simulink model "swpwmctrl"  (Simulink 7.0)
settings: Solver=ode1  StartTime=0.0  StopTime=4  FixedStep=0.0002  RelTol=1e-3
undefined symbols (not defined in the file or in its folder): Model_626, Sensoray
libraries: rtwinlib x6, simulink x6, dsparch4 x5, dspsigops x2, dspswit3 x2
settings Model: Creator=user  LastModifiedBy=user_2  SimulationMode=external  ExtModeTrigDuration=60000  BufferReuse=off
settings SolverCC: PositivePriorityOrder=on
settings DataIOCC: MaxDataPoints=60000
settings OptimizationCC: BooleanDataType=off  InlineInvariantSignals=on  OptimizeBlockIOStorage=off  BufferReuse=off  ExpressionFolding=off  LocalBlockOutputs=off
settings HardwareCC: TargetEndianess=LittleEndian  TargetHWDeviceType=MATLAB Host
settings RTWCC: SystemTargetFile=rtwin.tlc  TemplateMakefile=rtwin.tmf  Description=Real-Time Windows Target  ProcessScript=rtwin_make_rtw_hook
settings RTWinTargetCC: GenFloatMathFcnCalls=ANSI_C  ModelReferenceCompliant=off  CompOptLevelCompliant=off  PortableWordSizes=off  CCOptimize=on

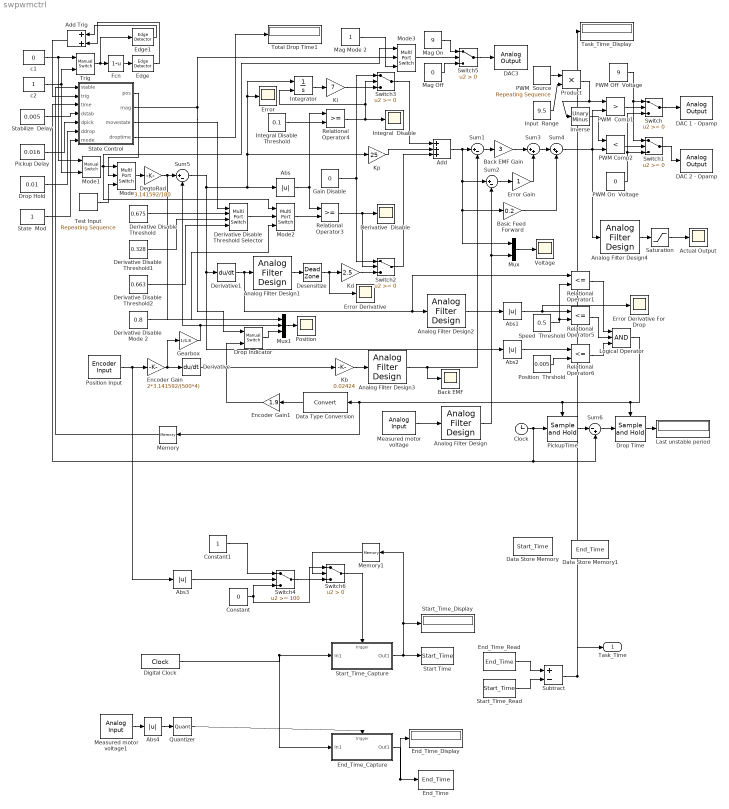
== system swpwmctrl ==
  Abs{,1..4} (5 alike) : Abs  OutDataType=sfix(16)  OutScaling=2^0
  Actual Output : Scope
      settings: YMin=-15  YMax=15  SaveName=ScopeData4  MaxDataPoints=60000
  Add : Sum  Inputs=+++  OutDataType=sfix(16)  OutScaling=2^-10
  Add Trig : Sum  Orientation=left  OutDataType=sfix(16)  OutScaling=2^-10
  Analog Filter Design : dsparch4/Analog Filter Design  method=Butterworth  filttype=Lowpass  N=3  Wlo=100  Whi=80  Rp=2  Rs=40
  Analog Filter Design1 : dsparch4/Analog Filter Design  method=Butterworth  filttype=Lowpass  N=3  Wlo=100  Whi=80  Rp=2  Rs=40
  Analog Filter Design2 : dsparch4/Analog Filter Design  method=Butterworth  filttype=Lowpass  N=3  Wlo=80  Whi=80  Rp=2  Rs=40
  Analog Filter Design3 : dsparch4/Analog Filter Design  method=Butterworth  filttype=Lowpass  N=3  Wlo=100  Whi=80  Rp=2  Rs=40
  Analog Filter Design4 : dsparch4/Analog Filter Design  method=Butterworth  filttype=Lowpass  N=3  Wlo=85  Whi=80  Rp=2  Rs=40
  Back EMF : Scope
      settings: YMin=-1  YMax=1  SaveName=ScopeData10  MaxDataPoints=60000
  Back EMF Gain : Gain  Gain=3  ParameterDataType=sfix(16)  ParameterScaling=2^0  OutDataType=sfix(16)  OutScaling=2^0
  Basic Feed  Forward : Gain  Gain=0.2  ParameterDataType=sfix(16)  ParameterScaling=2^0  OutDataType=sfix(16)  OutScaling=2^0
  Clock : Clock
      settings: Decimation=10
  Constant : Constant  Value=0  OutDataType=sfix(16)  OutScaling=2^0
  Constant1 : Constant  OutDataType=sfix(16)  OutScaling=2^0
  DAC 1 - Opamp : rtwinlib/Analog Output  SampleTime=-1  DrvName=Sensoray/Model_626  DrvAddress=4294967295  DrvOptions=zeros(1,0)  Channels=1  RangeMode=1  VoltRange=1  InitialValue=[]  FinalValue=[]
      settings: AttributesFormatString=Sensoray\nModel 626 [auto]
  DAC 2 - Opamp : rtwinlib/Analog Output  SampleTime=-1  DrvName=Sensoray/Model_626  DrvAddress=4294967295  DrvOptions=zeros(1,0)  Channels=2  RangeMode=1  VoltRange=1  InitialValue=[]  FinalValue=[]
      settings: AttributesFormatString=Sensoray\nModel 626 [auto]
  DAC3 : rtwinlib/Analog Output  SampleTime=-1  DrvName=Sensoray/Model_626  DrvAddress=4294967295  DrvOptions=zeros(1,0)  Channels=3  RangeMode=1  VoltRange=1  InitialValue=[]  FinalValue=[]
      settings: AttributesFormatString=Sensoray\nModel 626 [auto]
  Data Store Memory : DataStoreMemory  DataStoreName=Start_Time  ReadBeforeWriteMsg=warning  WriteAfterWriteMsg=warning  WriteAfterReadMsg=warning  OutDataType=sfix(16)  OutScaling=2^0
  Data Store Memory1 : DataStoreMemory  DataStoreName=End_Time  ReadBeforeWriteMsg=warning  WriteAfterWriteMsg=warning  WriteAfterReadMsg=warning  OutDataType=sfix(16)  OutScaling=2^0
  Data Type Conversion : DataTypeConversion  Orientation=left  OutDataTypeMode=double  OutDataType=sfix(16)  OutScaling=2^0
  DegtoRad : Gain  Gain=3.141592/180  ParameterDataType=sfix(16)  ParameterScaling=2^0  OutDataType=sfix(16)  OutScaling=2^0
  Derivative : Derivative
  Derivative  Disable : Scope
      settings: YMin=-0.25  YMax=3.25  SaveName=ScopeData3  MaxDataPoints=60000
  Derivative Disable Mode 2 : Constant  Value=0.8  OutDataType=sfix(16)  OutScaling=2^0
  Derivative Disable Threshold : Constant  Value=0.675  OutDataType=sfix(16)  OutScaling=2^0
  Derivative Disable Threshold Selector : MultiPortSwitch  Inputs=3  zeroidx=on  OutDataType=sfix(16)  OutScaling=2^0
  Derivative Disable Threshold1 : Constant  Value=0.328  OutDataType=sfix(16)  OutScaling=2^0
  Derivative Disable Threshold2 : Constant  Value=0.663  OutDataType=sfix(16)  OutScaling=2^0
  Derivative1 : Derivative
  Desensitize : DeadZone  LowerValue=-0.1  UpperValue=0.1  SaturateOnIntegerOverflow=on
  Digital Clock : DigitalClock  SampleTime=-1
  Drop Hold : Constant  Value=0.01  OutDataType=sfix(16)  OutScaling=2^0
  Drop Indicator : simulink/Signal Routing/Manual Switch  SystemSampleTime=-1  sw=1  action=0  varsize=off
  Drop Time : dspsigops/Sample and Hold  SystemSampleTime=-1  trig=Rising edge  initCond=0  latchinput=off
  Edge : dspswit3/Edge Detector  SystemSampleTime=-1
  Edge1 : dspswit3/Edge Detector  SystemSampleTime=-1
  Encoder Gain : Gain  Gain=2*3.141592/(500*4)  ParameterDataType=sfix(16)  ParameterScaling=2^0  OutDataType=sfix(16)  OutScaling=2^0
  Encoder Gain1 : Gain  Orientation=left  Gain=1.9  ParameterDataType=sfix(16)  ParameterScaling=2^0  OutDataType=sfix(16)  OutScaling=2^0
  End_Time : DataStoreWrite  DataStoreName=End_Time  SampleTime=-1
  End_Time_Capture : Subsystem  TreatAsAtomicUnit=on
  End_Time_Display : Display
  End_Time_Read : DataStoreRead  DataStoreName=End_Time  SampleTime=0
  Error : Scope
      settings: YMin=-0.05  YMax=0.05  SaveName=ScopeData2  MaxDataPoints=60000
  Error Derivative : Scope
      settings: YMin=-1  YMax=1  SaveName=ScopeData8  MaxDataPoints=60000
  Error Derivative For Drop : Scope
      settings: YMin=0  YMax=2  SaveName=ScopeData9  MaxDataPoints=60000
  Error Gain : Gain  ParameterDataType=sfix(16)  ParameterScaling=2^0  OutDataType=sfix(16)  OutScaling=2^0
  Fcn : Fcn  Expr=1-u
  Gain Disable : Constant  Value=0  OutDataType=sfix(16)  OutScaling=2^0
  Gearbox : Gain  Gain=1/4.8  ParameterDataType=sfix(16)  ParameterScaling=2^0  OutDataType=sfix(16)  OutScaling=2^0
  Input  Range : Constant  Value=9.5  OutDataType=sfix(16)  OutScaling=2^0
  Integral  Disable : Scope
      settings: YMin=-0.25  YMax=3.25  SaveName=ScopeData5  MaxDataPoints=60000
  Integral Disable Threshold : Constant  Value=0.1  OutDataType=sfix(16)  OutScaling=2^0
  Integrator : Integrator  ExternalReset=falling
  Inverse : simulink/Math Operations/Unary Minus  DoSatur=off
  Kb : Gain  Gain=0.02424  ParameterDataType=sfix(16)  ParameterScaling=2^0  OutDataType=sfix(16)  OutScaling=2^0
  Kd : Gain  Gain=2.5  ParameterDataType=sfix(16)  ParameterScaling=2^0  OutDataType=sfix(16)  OutScaling=2^0
  Ki : Gain  Gain=7  ParameterDataType=sfix(16)  ParameterScaling=2^0  OutDataType=sfix(16)  OutScaling=2^0
  Kp : Gain  Gain=25  ParameterDataType=sfix(16)  ParameterScaling=2^0  OutDataType=sfix(16)  OutScaling=2^0
  Last unstable period : Display
  Logical Operator : Logic  Inputs=3  AllPortsSameDT=off  OutDataTypeMode=boolean
  Mag Mode 2 : Constant  OutDataType=sfix(16)  OutScaling=2^0
  Mag Off : Constant  Value=0  OutDataType=sfix(16)  OutScaling=2^0
  Mag On : Constant  Value=9  OutDataType=sfix(16)  OutScaling=2^0
  Measured motor voltage : rtwinlib/Analog Input  SampleTime=-1  DrvName=Sensoray/Model_626  DrvAddress=4294967295  DrvOptions=zeros(1,0)  Channels=1  RangeMode=1  VoltRange=1  DataType=1
      settings: AttributesFormatString=Sensoray\nModel 626 [auto]
  Measured motor voltage1 : rtwinlib/Analog Input  SampleTime=-1  DrvName=Sensoray/Model_626  DrvAddress=4294967295  DrvOptions=zeros(1,0)  Channels=2  RangeMode=1  VoltRange=1  DataType=1
      settings: AttributesFormatString=Sensoray\nModel 626 [auto]
  Memory : Memory  Orientation=left
  Memory1 : Memory  Orientation=left
  Mode : MultiPortSwitch  Inputs=2  zeroidx=on  OutDataType=sfix(16)  OutScaling=2^0
  Mode1 : simulink/Signal Routing/Manual Switch  SystemSampleTime=-1  sw=1  action=0  varsize=off
  Mode2 : MultiPortSwitch  Inputs=2  zeroidx=on  OutDataType=sfix(16)  OutScaling=2^0
  Mode3 : MultiPortSwitch  Inputs=2  zeroidx=on  OutDataType=sfix(16)  OutScaling=2^0
  Mux : Mux  Inputs=2
  Mux1 : Mux  Inputs=3
  PWM Comp2 : RelationalOperator  Operator=<  LogicOutDataTypeMode=boolean
  PWM  Comp1 : RelationalOperator  Operator=>  LogicOutDataTypeMode=boolean
  PWM  Source : simulink/Sources/Repeating Sequence  SystemSampleTime=-1  rep_seq_t=[0 0.01]  rep_seq_y=[0 1]
  PWM Off  Voltage : Constant  Value=9  OutDataType=sfix(16)  OutScaling=2^0
  PWM On  Voltage : Constant  Value=0  OutDataType=sfix(16)  OutScaling=2^0
  Pickup Delay : Constant  Value=0.016  OutDataType=sfix(16)  OutScaling=2^0
  PickupTime : dspsigops/Sample and Hold  SystemSampleTime=-1  trig=Falling edge  initCond=0  latchinput=off
  Position : Scope
      settings: YMin=-2  YMax=1.2  MaxDataPoints=60000
  Position  Thrshold : Constant  Value=0.005  OutDataType=sfix(16)  OutScaling=2^0
  Position Input : rtwinlib/Encoder Input  SampleTime=-1  DrvName=Sensoray/Model_626  DrvAddress=4294967295  DrvOptions=zeros(1,0)  Channels=[4]  QuadMode=3  IndexPulse=2  InputFilter=Inf  DataType=1
      settings: AttributesFormatString=Sensoray\nModel 626 [auto]
  Product : Product  OutDataType=sfix(16)  OutScaling=2^0  RndMeth=Zero
  Quantizer : Quantizer
  Relational Operator1 : RelationalOperator  Operator=<=  LogicOutDataTypeMode=boolean
  Relational Operator3 : RelationalOperator  LogicOutDataTypeMode=boolean
  Relational Operator4 : RelationalOperator  LogicOutDataTypeMode=boolean
  Relational Operator5 : RelationalOperator  Operator=<=  LogicOutDataTypeMode=boolean
  Relational Operator6 : RelationalOperator  Operator=<=  LogicOutDataTypeMode=boolean
  Saturation : Saturate  UpperLimit=10  LowerLimit=-10  OutDataType=sfix(16)  OutScaling=2^0
  Speed  Threshold : Constant  Value=0.5  OutDataType=sfix(16)  OutScaling=2^0
  Stabilize  Delay : Constant  Value=0.005  OutDataType=sfix(16)  OutScaling=2^0
  Start Time : DataStoreWrite  DataStoreName=Start_Time  SampleTime=-1
  Start_Time_Capture : Subsystem  TreatAsAtomicUnit=on
  Start_Time_Display : Display
  Start_Time_Read : DataStoreRead  DataStoreName=Start_Time  SampleTime=0
  State  Mod : Constant  OutDataType=sfix(16)  OutScaling=2^0
  State Control : Stateflow chart
  Subtract : Sum  Inputs=+-  OutDataType=sfix(16)  OutScaling=2^-10
  Sum1 : Sum  Inputs=|+-  OutDataType=sfix(16)  OutScaling=2^0
  Sum2 : Sum  Inputs=|+-  OutDataType=sfix(16)  OutScaling=2^0
  Sum3 : Sum  Inputs=|++  OutDataType=sfix(16)  OutScaling=2^0
  Sum4 : Sum  Inputs=|++  OutDataType=sfix(16)  OutScaling=2^0
  Sum5 : Sum  Inputs=|+-  OutDataType=sfix(16)  OutScaling=2^0
  Sum6 : Sum  Inputs=|-+  OutDataType=sfix(16)  OutScaling=2^0
  Switch{,1..3} (4 alike) : Switch  OutDataType=sfix(16)  OutScaling=2^0
  Switch4 : Switch  Threshold=100  OutDataType=sfix(16)  OutScaling=2^0
  Switch5 : Switch  Criteria=u2 > Threshold  OutDataType=sfix(16)  OutScaling=2^0
  Switch6 : Switch  Criteria=u2 > Threshold  OutDataType=sfix(16)  OutScaling=2^0
  Task_Time_Display : Display
  Test Input : simulink/Sources/Repeating Sequence  SystemSampleTime=-1  rep_seq_t=[0 1 1.01 4 4.01 5]  rep_seq_y=[0 0 90 90 0 0]
  Total Drop Time1 : Display
  Trig : simulink/Signal Routing/Manual Switch  SystemSampleTime=-1  sw=0  action=0  varsize=off
  Voltage : Scope
      settings: YMin=-9  YMax=9  MaxDataPoints=60000
  c1 : Constant  Value=0  OutDataType=sfix(16)  OutScaling=2^0
  c2 : Constant  OutDataType=sfix(16)  OutScaling=2^0
  Task_Time : Outport  OutDataType=sfix(16)  OutScaling=2^0
  wires:
  PWM  Comp1/1 -> Switch/2
  Switch/1 -> DAC 1 - Opamp/1
  PWM Off  Voltage/1 -> Switch/1, Switch1/1
  PWM Comp2/1 -> Switch1/2
  PWM On  Voltage/1 -> Switch1/3, Switch/3
  Product/1 -> PWM  Comp1/1, Inverse/1
  PWM  Source/1 -> Product/1
  Input  Range/1 -> Product/2
  Switch1/1 -> DAC 2 - Opamp/1
  Measured motor voltage/1 -> Analog Filter Design/1
  Position Input/1 -> Encoder Gain/1, Abs3/1
  Encoder Gain/1 -> Derivative/1, Gearbox/1
  Derivative/1 -> Kb/1
  Add/1 -> Sum2/1, Mux/1, Basic Feed  Forward/1, Sum1/1
  Sum1/1 -> Back EMF Gain/1
  Kb/1 -> Analog Filter Design3/1
  Sum2/1 -> Error Gain/1
  Back EMF Gain/1 -> Sum3/1
  Error Gain/1 -> Sum3/2
  Inverse/1 -> PWM Comp2/1
  Analog Filter Design/1 -> Sum2/2, Mux/2
  Mux/1 -> Voltage/1
  Sum4/1 -> PWM Comp2/2, PWM  Comp1/2, Analog Filter Design4/1
  Sum3/1 -> Sum4/1
  Basic Feed  Forward/1 -> Sum4/2
  DegtoRad/1 -> Sum5/1, Mux1/1
  Sum5/1 -> Derivative1/1, Abs2/1, Abs/1, Error/1, Integrator/1, Kp/1
  Gearbox/1 -> Sum5/2, Mux1/2
  Derivative1/1 -> Analog Filter Design1/1, Analog Filter Design2/1, Relational Operator1/1
  Kp/1 -> Add/2
  Integrator/1 -> Ki/1
  Gain Disable/1 -> Switch2/1, Switch3/1
  Relational Operator3/1 -> Switch2/2, Derivative  Disable/1
  Mux1/1 -> Position/1
  Abs/1 -> Relational Operator3/1, Relational Operator4/1
  Kd/1 -> Switch2/3
  Switch2/1 -> Add/3
  Switch3/1 -> Add/1
  Ki/1 -> Switch3/3
  Integral Disable Threshold/1 -> Relational Operator4/2
  Relational Operator4/1 -> Switch3/2, Integrator/2, Integral  Disable/1
  Analog Filter Design1/1 -> Desensitize/1
  Logical Operator/1 -> Drop Time/Trigger, PickupTime/Trigger, Data Type Conversion/1, Memory/1
  Switch5/1 -> DAC3/1
  Mag On/1 -> Switch5/1
  Mag Off/1 -> Switch5/3
  Relational Operator6/1 -> Logical Operator/3
  Relational Operator5/1 -> Logical Operator/2
  Position  Thrshold/1 -> Relational Operator6/2
  Abs1/1 -> Relational Operator5/1, Error Derivative For Drop/1
  Abs2/1 -> Relational Operator6/1
  Analog Filter Design2/1 -> Abs1/1
  Data Type Conversion/1 -> Encoder Gain1/1
  Clock/1 -> PickupTime/1, Sum6/2, State Control/3(time)
  PickupTime/1 -> Sum6/1
  Sum6/1 -> Drop Time/1
  Drop Time/1 -> Last unstable period/1
  Analog Filter Design3/1 -> Sum1/2, Back EMF/1
  Desensitize/1 -> Kd/1, Error Derivative/1
  Derivative Disable Threshold/1 -> Derivative Disable Threshold Selector/2
  Derivative Disable Threshold1/1 -> Derivative Disable Threshold Selector/3
  State Control/3(movestate) -> Derivative Disable Threshold Selector/1
  Trig/1 -> Edge1/1, Fcn/1
  c1/1 -> Trig/1, Mode1/1
  c2/1 -> Trig/2, Mode1/2
  Memory/1 -> State Control/1(stable)
  Fcn/1 -> Edge/1
  Mode/1 -> DegtoRad/1
  Mode1/1 -> Mode3/1, Mode/1, Mode2/1
  State Control/1(pos) -> Mode/2
  Test Input/1 -> Mode/3
  Derivative Disable Threshold Selector/1 -> Mode2/2
  Mode2/1 -> Relational Operator3/2
  Derivative Disable Mode 2/1 -> Mode2/3
  Mode3/1 -> Switch5/2
  State Control/2(mag) -> Mode3/2, Drop Indicator/1
  Mag Mode 2/1 -> Mode3/3
  State Control/4(droptime) -> Total Drop Time1/1
  Edge1/1 -> Add Trig/1
  Edge/1 -> Add Trig/2
  Add Trig/1 -> State Control/2(trig)
  Stabilize  Delay/1 -> State Control/4(dstab)
  Pickup Delay/1 -> State Control/5(dpick)
  Drop Hold/1 -> State Control/6(ddrop)
  Analog Filter Design4/1 -> Saturation/1
  Drop Indicator/1 -> Mux1/3
  Encoder Gain1/1 -> Drop Indicator/2
  Saturation/1 -> Actual Output/1
  Speed  Threshold/1 -> Relational Operator1/2, Relational Operator5/2
  Relational Operator1/1 -> Logical Operator/1
  State  Mod/1 -> State Control/7(mode)
  Derivative Disable Threshold2/1 -> Derivative Disable Threshold Selector/4
  Measured motor voltage1/1 -> Abs4/1
  Digital Clock/1 -> Start_Time_Capture/1(In1), End_Time_Capture/1(In1)
  Constant/1 -> Switch4/3, Switch6/1
  Constant1/1 -> Switch4/1
  End_Time_Read/1 -> Subtract/1
  Quantizer/1 -> End_Time_Capture/Trigger
  End_Time_Capture/1(Out1) -> End_Time/1, End_Time_Display/1
  Start_Time_Read/1 -> Subtract/2
  Subtract/1 -> Task_Time_Display/1, Task_Time/1
  Abs3/1 -> Switch4/2
  Abs4/1 -> Quantizer/1
  Start_Time_Capture/1(Out1) -> Start Time/1, Start_Time_Display/1, Memory1/1
  Switch6/1 -> Start_Time_Capture/Trigger
  Memory1/1 -> Switch6/2
  Switch4/1 -> Switch6/3

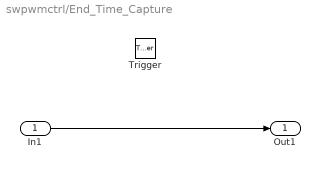
== system swpwmctrl/End_Time_Capture ==
  In1 : Inport  OutDataType=sfix(16)  OutScaling=2^0
  Trigger : TriggerPort
  Out1 : Outport  OutDataType=sfix(16)  OutScaling=2^0
  wires:
  In1/1 -> Out1/1

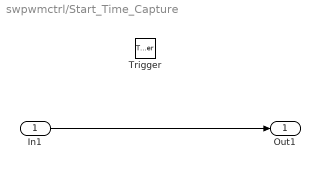
== system swpwmctrl/Start_Time_Capture ==
  In1 : Inport  OutDataType=sfix(16)  OutScaling=2^0
  Trigger : TriggerPort
  Out1 : Outport  OutDataType=sfix(16)  OutScaling=2^0
  wires:
  In1/1 -> Out1/1

== matlab function State Control ==
  data: stable input inherited; pos output inherited; trig input inherited; mag output inherited; movestate output inherited; time input inherited; droptime output inherited; dstab input inherited; dpick input inherited; ddrop input inherited; mode input inherited
function [pos,mag,movestate,droptime] = fcn(stable, trig, time,dstab,dpick,ddrop,mode)
% This block supports the Embedded MATLAB subset.
% See the help menu for details. 

persistent state;
persistent delayuntill;
persistent skipnext;

persistent startdrop;
persistent lastdroptime;

persistent lastpos;
persistent lastmag;
persistent lastmovestate;

if isempty(state)
   state = 0;
   delayuntill = 0;
   lastpos = 0;
   lastmag = 0;
   lastmovestate = 0;
   skipnext = false;
   startdrop = 0;
   lastdroptime = 0;
end

pos = lastpos;
mag = lastmag;
movestate = lastmovestate;
droptime = lastdroptime;

if (time < delayuntill) || skipnext
    skipnext = false;
    %statedbg = state;
    return
end

laststate = state;

% Standard
if mode == 0
switch state
    case 0
        % Wait for user to trigger start
        pos = 0;
        mag = 0;
        movestate = 0;
        if trig
            state = state + 1;
            pos = 90;
            %skipnext = true;
        end
    case 1
        % Move to 90 then wait 
        if trig && stable
            state = state + 2;
            pos = 45;
            movestate = 1; 
            %skipnext = true;
        end
    case 3
        % Move to 45 then wait for manual trigger
        pos = 45;
        movestate = 1; 
        if stable && trig
            state = state + 1 ;
            pos = 90;
            %skipnext = true;
            startdrop = time;
        end
    case 4
        % Move to 90 then wait 
        if stable
            state = state + 1 ;
            delayuntill = time + dstab;
        end
    case 5
        % Pickup mag then wait
        if stable
            mag = 1;
            movestate = 0;    
            state = state + 1 ;
            delayuntill = time + dpick;
        end
    case 6
        % Start move to 0
        pos = 0;
        state = state + 1 ;
        %skipnext = true;
    case 7
        % Move to 0, drop and wait
        if stable
            state = state + 1 ;
            mag = 0;
            delayuntill = time + ddrop;
            lastdroptime = time - startdrop;
        end
    case 8
        % Repeat
        pos = 45;
        mag = 0;
        movestate = 1;
        state = 3;
        %skipnext = true;
    otherwise
        state = 0;
end

% Competition - 45 -> 90 -> 0
elseif mode == 1
switch state
    case 0
        % Start up
        pos = 0;
        mag = 0;
        movestate = 1;
        state = state + 1;
        delayuntill = time + 1;
    case 1
        % Go to pickup
        pos = 45;
        state = state + 1;
        %skipnext = true;
    case 2
        % Wait for additional stable time 
        if stable
            state = state + 1 ;
            delayuntill = time + dstab;
        end
    case 3
        %Pickup
        if stable
            state = state + 1 ;
            mag = 1;
            movestate = 0;
            %skipnext = true;
            delayuntill = time + dpick;
        end
    case 4
        % Move to drop
        movestate = 0;
        pos = -45;
        state = state + 1;
        %skipnext = true;
    case 5
        % drop
        if stable
            mag = 0;
            state = state + 1;
            delayuntill = time + ddrop;
            lastdroptime = time - 1;
        end
    case 6
        mag = 0;
        pos = 0;
        movestate = 1;
    otherwise
        state = 0;
end 

% Competition - 90 -> 0
elseif mode == 2
switch state
    case 0
        % Start up - wait for 1 second
        pos = 0;
        mag = 0;
        movestate = 2;
        state = state + 1;
        delayuntill = time + 1;
    case 1
        % Start up - get mag
        mag = 1;
        state = state + 1;
        delayuntill = time + dpick;
    case 2
        % Go to drop
        pos = -90;
        state = state + 1;
    case 3
        % Wait for additional stable time 
        if stable
            state = state + 1 ;
            mag = 0;
            delayuntill = time + ddrop;
            lastdroptime = time - 1;
        end
    case 4
        %End
        pos = 0;
        mag = 0;
        movestate = 0;
    otherwise
        state = 0;
end 
end

lastpos = pos;
lastmag = mag;
lastmovestate = movestate;
%statedbg = state;

if laststate ~= state
    skipnext = true;
end

droptime = lastdroptime;
